simulink model "Mode_Test"  (R2023b)
settings: Solver=FixedStepAuto  StartTime=0.0  StopTime=30  FixedStep=1e-3  RelTol=1e-3  EnableMultiTasking=on
undefined symbols (not defined in the file): D0, D1, PTC16, PTC17
libraries: frdmk64flib x6
settings Model: ExtModeTrigDuration=5  Creator=haley  LastModifiedBy=conno
settings OptimizationCC: EnhancedBackFolding=on  PassReuseOutputArgsAs=Individual arguments  ZeroExternalMemoryAtStartup=off  ZeroInternalMemoryAtStartup=off  MaxStackSize=64  OptimizeBlockOrder=speed  DifferentSizesBufferReuse=on  OptimizationCustomize=off  EfficientTunableParamExpr=on
settings DebuggingCC: ParameterTunabilityLossMsg=error
settings HardwareCC: ProdBitPerPointer=32  ProdBitPerSizeT=32  ProdBitPerPtrDiffT=32  ProdLargestAtomicInteger=Long  ProdLargestAtomicFloat=Double  ProdWordSize=32  ProdHWDeviceType=ARM Compatible->ARM Cortex
settings SFSimCC: MATLABDynamicMemAlloc=off
settings RTWCC: Description=Embedded Coder  SystemTargetFile=ert.tlc  HardwareBoard=NXP FRDM-K64F  TLCOptions="-aInlineSetEventsForThisBaseRateFcn=TLC_FALSE -aSuppressMultiTaskScheduler=TLC_FALSE  -aRateBasedStepFcn=0"  TemplateMakefile=ert_default_tmf  Toolchain=GNU Tools for ARM Embedded Processors
settings CodeAppCC: ForceParamTrailComments=on  IgnoreCustomStorageClasses=off  OperatorAnnotations=on  SimulinkDataObjDesc=on  SFDataObjDesc=on  InsertBlockDesc=on
settings ERTTargetCC: ExtModeTransport=4  ExtModeMexFile=sendToCommService

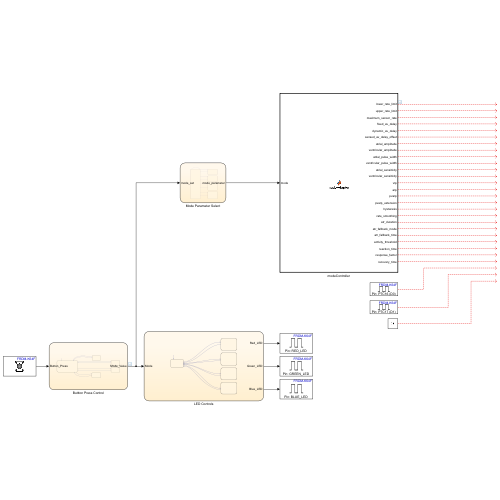
[thumbnail: Simulink's stored preview of the top-level diagram]
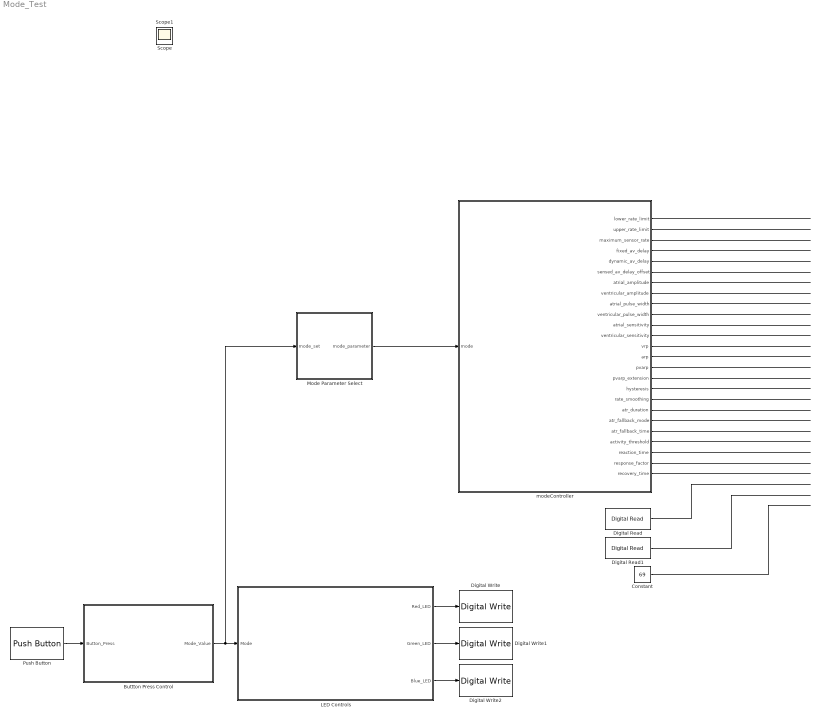
== system Mode_Test ==
  Buttton Press Control : Stateflow chart  TreatAsAtomicUnit=on
  Constant : Constant  Value=69
  Digital Read : frdmk64flib/Digital Read  Whichpin=PTC16 (D0)  SampleTime=-1
  Digital Read1 : frdmk64flib/Digital Read  Whichpin=PTC17 (D1)  SampleTime=-1
  Digital Write : frdmk64flib/Digital Write  Whichpin=RED_LED
  Digital Write1 : frdmk64flib/Digital Write  Whichpin=GREEN_LED
  Digital Write2 : frdmk64flib/Digital Write  Whichpin=BLUE_LED
  LED Controls : Stateflow chart  TreatAsAtomicUnit=on
  Mode Parameter Select : Stateflow chart  TreatAsAtomicUnit=on
  Push Button : frdmk64flib/Push Button  Whichswitch=SW3  SampleTime1=-1
  modeController : MATLAB Function  TreatAsAtomicUnit=on
  Scope : Scope
  Scope1 : Scope
  wires:
  LED Controls/3(Blue_LED) -> Digital Write2/1
  modeController/3(maximum_sensor_rate) -> ?
  Push Button/1 -> Buttton Press Control/1(Button_Press)
  Buttton Press Control/1(Mode_Value) -> Mode Parameter Select/1(mode_set), LED Controls/1(Mode)
  modeController/1(lower_rate_limit) -> ?
  modeController/18(rate_smoothing) -> ?
  LED Controls/1(Red_LED) -> Digital Write/1
  Mode Parameter Select/1(mode_parameter) -> modeController/1(mode)
  LED Controls/2(Green_LED) -> Digital Write1/1
  modeController/2(upper_rate_limit) -> ?
  modeController/4(fixed_av_delay) -> ?
  modeController/5(dynamic_av_delay) -> ?
  modeController/6(sensed_av_delay_offset) -> ?
  modeController/7(atrial_amplitude) -> ?
  Digital Read1/1 -> ?
  modeController/8(ventricular_amplitude) -> ?
  Digital Read/1 -> ?
  modeController/9(atrial_pulse_width) -> ?
  modeController/16(pvarp_extension) -> ?
  modeController/10(ventricular_pulse_width) -> ?
  modeController/21(atr_fallback_time) -> ?
  modeController/11(atrial_sensitivity) -> ?
  modeController/24(response_factor) -> ?
  modeController/12(ventricular_sensitivity) -> ?
  modeController/13(vrp) -> ?
  modeController/14(arp) -> ?
  modeController/15(pvarp) -> ?
  modeController/17(hysteresis) -> ?
  modeController/19(atr_duration) -> ?
  modeController/20(atr_fallback_mode) -> ?
  modeController/22(activity_threshold) -> ?
  modeController/23(reaction_time) -> ?
  modeController/25(recovery_time) -> ?
  Constant/1 -> ?

== matlab function Mode_Test/modeController ==
  data: mode input; lower_rate_limit output; upper_rate_limit output; maximum_sensor_rate output; fixed_av_delay output; dynamic_av_delay output; sensed_av_delay_offset output; atrial_amplitude output; ventricular_amplitude output; atrial_pulse_width output; ventricular_pulse_width output; atrial_sensitivity output; ventricular_sensitivity output; vrp output; arp output; pvarp output; pvarp_extension output; hysteresis output; rate_smoothing output; atr_duration output; atr_fallback_mode output; atr_fallback_time output; activity_threshold output; reaction_time output; response_factor output; recovery_time output
function [lower_rate_limit, upper_rate_limit, maximum_sensor_rate, fixed_av_delay, dynamic_av_delay, sensed_av_delay_offset, atrial_amplitude, ventricular_amplitude, atrial_pulse_width, ventricular_pulse_width, atrial_sensitivity, ventricular_sensitivity, vrp, arp, pvarp, pvarp_extension, hysteresis, rate_smoothing, atr_duration, atr_fallback_mode, atr_fallback_time, activity_threshold, reaction_time, response_factor, recovery_time] = modeAdapter(mode)
    
    
    % Start by taking the mode input as a binary number, and extrapolating
    % all the active parameters.
    % Should return 1 if true and 0 if false
    %mode_vector = num2str(mode) - '0'; %convert the input to a list
    %N = 1994;
    mode_vector = zeros(1,25);
    i=1;
    while mode > 0
      data = mod(mode,2);
      mode_vector(26-i) = data; %ok
      mode = (mode-data)/10;
      i = i+1;
    end

    
    lower_rate_limit = mode_vector(1); %Parameter 1
    upper_rate_limit = mode_vector(2); %Parameter 2
    maximum_sensor_rate = mode_vector(3); %Parameter 3
    fixed_av_delay = mode_vector(4); %Parameter 4
    dynamic_av_delay = mode_vector(5); %Parameter 5
    sensed_av_delay_offset = mode_vector(6); %Parameter 6
    atrial_amplitude = mode_vector(7); %Parameter 7
    ventricular_amplitude = mode_vector(8); %Parameter 8
    atrial_pulse_width = mode_vector(9); %Parameter 9
    ventricular_pulse_width = mode_vector(10); %Parameter 10
    atrial_sensitivity = mode_vector(11); %Parameter 11
    ventricular_sensitivity = mode_vector(12); %Parameter 12
    vrp = mode_vector(13); %Parameter 13
    arp = mode_vector(14); %Parameter 14
    pvarp = mode_vector(15); %Parameter 15
    pvarp_extension = mode_vector(16); %Parameter 16
    hysteresis = mode_vector(17); %Parameter 17
    rate_smoothing = mode_vector(18); %Parameter 18
    atr_duration = mode_vector(19); %Parameter 19
    atr_fallback_mode = mode_vector(20); %Parameter 20
    atr_fallback_time = mode_vector(21); %Parameter 21
    activity_threshold = mode_vector(22); %Parameter 22
    reaction_time = mode_vector(23); %Parameter 23
    response_factor = mode_vector(24); %Parameter 24
    recovery_time = mode_vector(25); %Parameter 25

    set_lower_rate_limit = (40); %Parameter 1
    set_upper_rate_limit = (100); %Parameter 2
    set_maximum_sensor_rate = (100); %Parameter 3
    set_fixed_av_delay = (100); %Parameter 4
    set_dynamic_av_delay = (1); %Parameter 5
    set_sensed_av_delay_offset = (-50); %Parameter 6
    set_atrial_amplitude = (2.5); %Parameter 7
    set_ventricular_amplitude = (2.5); %Parameter 8
    set_atrial_pulse_width = (0.05); %Parameter 9
    set_ventricular_pulse_width = (0.05); %Parameter 10
    set_atrial_sensitivity = (0.5); %Parameter 11
    set_ventricular_sensitivity = (0.5); %Parameter 12
    set_vrp = (300); %Parameter 13
    set_arp = (300); %Parameter 14
    set_pvarp = (300); %Parameter 15
    set_pvarp_extension = (200); %Parameter 16
    set_hysteresis = (set_lower_rate_limit); %Parameter 17
    set_rate_smoothing = (15); %Parameter 18
    set_atr_duration = (10); %Parameter 19
    set_atr_fallback_mode = (1); %Parameter 20
    set_atr_fallback_time = (3); %Parameter 21
    set_activity_threshold = (3); %Parameter 22
    set_reaction_time = (30); %Parameter 23
    set_response_factor = (10); %Parameter 24
    set_recovery_time = (10); %Parameter 25
    
    length = 25;
    
    input_list = [lower_rate_limit, upper_rate_limit, maximum_sensor_rate, fixed_av_delay, dynamic_av_delay, sensed_av_delay_offset, atrial_amplitude, ventricular_amplitude, atrial_pulse_width, ventricular_pulse_width, atrial_sensitivity, ventricular_sensitivity, vrp, arp, pvarp, pvarp_extension, hysteresis, rate_smoothing, atr_duration, atr_fallback_mode, atr_fallback_time, activity_threshold, reaction_time, response_factor, recovery_time];
    parameter_list = [set_lower_rate_limit, set_upper_rate_limit, set_maximum_sensor_rate, set_fixed_av_delay, set_fixed_av_delay, set_dynamic_av_delay, set_sensed_av_delay_offset, set_atrial_amplitude, set_ventricular_amplitude, set_atrial_pulse_width, set_ventricular_pulse_width, set_atrial_sensitivity, set_ventricular_sensitivity, set_vrp, set_arp, set_pvarp, set_pvarp_extension, set_hysteresis, set_rate_smoothing, set_atr_duration, set_atr_fallback_mode, set_atr_fallback_time, set_activity_threshold, set_reaction_time, set_response_factor, set_recovery_time];
    
    for i = 1:length
        if input_list(i) == 1
            input_list(i) = parameter_list(i);
        end
    end
    
    %Redeclare the values
    lower_rate_limit = input_list(1); %Parameter 1
    upper_rate_limit = input_list(2); %Parameter 2
    maximum_sensor_rate = input_list(3); %Parameter 3
    fixed_av_delay = input_list(4); %Parameter 4
    dynamic_av_delay = input_list(5); %Parameter 5
    sensed_av_delay_offset = input_list(6); %Parameter 6
    atrial_amplitude = input_list(7); %Parameter 7
    ventricular_amplitude = input_list(8); %Parameter 8
    atrial_pulse_width = input_list(9); %Parameter 9
    ventricular_pulse_width = input_list(10); %Parameter 10
    atrial_sensitivity = input_list(11); %Parameter 11
    ventricular_sensitivity = input_list(12); %Parameter 12
    vrp = input_list(13); %Parameter 13
    arp = input_list(14); %Parameter 14
    pvarp = input_list(15); %Parameter 15
    pvarp_extension = input_list(16); %Parameter 16
    hysteresis = input_list(17); %Parameter 17
    rate_smoothing = input_list(18); %Parameter 18
    atr_duration = input_list(19); %Parameter 19
    atr_fallback_mode = input_list(20); %Parameter 20
    atr_fallback_time = input_list(21); %Parameter 21
    activity_threshold = input_list(22); %Parameter 22
    reaction_time = input_list(23); %Parameter 23
    response_factor = input_list(24); %Parameter 24
    recovery_time = input_list(25); %Parameter 25
    
    
end

== stateflow chart Mode_Test/Mode Parameter Select ==
  state OFF
    % Launch Point for determining mode, takes input
    % and selects proper functionality
    % if no mode selected (MODE 0), wait for it to change
  state AOO
    entry:
    %{
    Parameters Needed:
    LRL
    URL
    Atrial Amplitude
    Atrial Pulse Width
    %}
    mode_parameter = 0b1100001010000000000000000;
  state VOO
    entry:
    %{
    Parameters Needed:
    LRL
    URL
    Ventricular Amplitude
    Ventricular Pulse Width
    %}
    mode_parameter = 0b1100000101000000000000000;
  state AAI
    entry:
    %{
    Parameters Needed:
    Lower Rate Limit
    Upper Rate Limit
    Atrial Amplitude
    Atrial Pulse Width
    Hysteresis
    Rate Smoothing
    Atrial Sensitivity
    ARP
    PVARP
    %}
    mode_parameter = 0b1100001010100110110000000;
  state VVI
    entry:
    %{
    Parameters Needed:
    LRL
    URL
    Ventricle Amplitude
    Ventricle Pulse Width
    Hysteresis
    Rate Smoothing
    Ventricular Sensitivity
    VRP
    %}
    mode_parameter = 0b1100000101011000110000000;
  OFF -> OFF [order 1] : [mode_set == 0]
  OFF -> AOO [order 2] : [mode_set == 1]
  AOO -> OFF
  OFF -> VOO [order 3] : [mode_set == 2]
  VOO -> OFF
  OFF -> AAI [order 4] : [mode_set == 3]
  (default) -> OFF
  AAI -> OFF
  OFF -> VVI [order 5] : [mode_set == 4]
  VVI -> OFF
  data: mode_parameter output; mode_set input

== stateflow chart Mode_Test/LED Controls ==
  state AOO
    entry:
    Red_LED = 1
    Green_LED = 0
    Blue_LED = 1
  state VOO
    entry:
    Red_LED = 0
    Green_LED = 1
    Blue_LED = 0
  state Controller
  state AAI
    entry:
    Red_LED = 0
    Green_LED = 0
    Blue_LED = 1
  state VVI
    entry:
    Red_LED = 1
    Green_LED = 0
    Blue_LED = 0
  Controller -> AOO [order 1] : [Mode == 1]
  AOO -> Controller
  (default) -> Controller
  Controller -> VOO [order 2] : [Mode == 2]
  VOO -> Controller
  Controller -> AAI [order 3] : [Mode == 3]
  AAI -> Controller
  Controller -> VVI [order 4] : [Mode == 4]
  VVI -> Controller
  data: Mode input; Red_LED output; Green_LED output; Blue_LED output

== stateflow chart Mode_Test/Buttton Press Control ==
  state AOO
    entry:
    Mode_Value = 1
  state VOO
    entry:
    Mode_Value = 2
  state Controller
    entry:
    counter = 1 + mod(counter,4) %mod  4
  state AAI
    entry:
    Mode_Value = 3
  state VVI
    entry:
    Mode_Value = 4
  AOO -> Controller : [Button_Press == 0]
  Controller -> AOO [order 1] : [Button_Press == 1 && counter == 1]
  (default) -> Controller
  Controller -> VOO [order 2] : [Button_Press  == 1 && counter == 2]
  VOO -> Controller : [Button_Press  == 0]
  Controller -> AAI [order 3] : [Button_Press  == 1 && counter == 3]
  AAI -> Controller : [Button_Press  == 0]
  VVI -> Controller : [Button_Press  == 0]
  Controller -> VVI [order 4] : [Button_Press  == 1 && counter == 4]
  data: Mode_Value output; Button_Press input; counter local =0
